simulink model "Modelo_Tanque_Malha_Aberta"  (R2022a)
settings: Solver=FixedStepAuto  StartTime=0.0  StopTime=2500  FixedStep=1e-3  RelTol=1e-3
libraries: simulink x1
settings Model: Creator=User  LastModifiedBy=User
settings DebuggingCC: UnconnectedInputMsg=warning  UnconnectedOutputMsg=warning  UnconnectedLineMsg=warning
settings RTWCC: DLArmComputeVersion=19.05

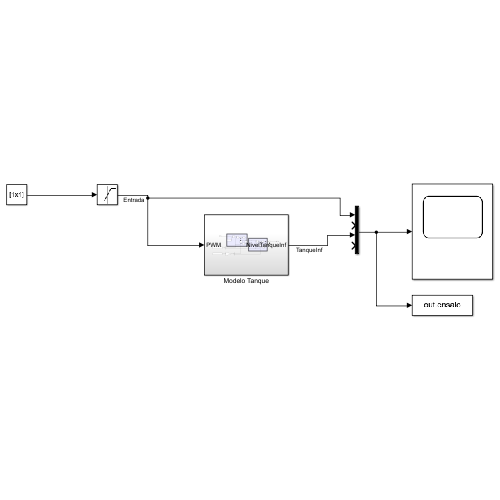
[thumbnail: Simulink's stored preview of the top-level diagram]
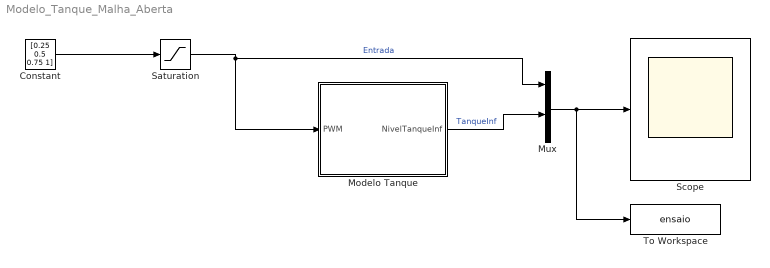
== system Modelo_Tanque_Malha_Aberta ==
  Constant : Constant  Value=[0.25 0.5 0.75 1]
  Modelo Tanque : Subsystem
  Mux : Mux
  Saturation : Saturate  UpperLimit=1  LowerLimit=0
  Scope : Scope
  To Workspace : ToWorkspace  VariableName=ensaio  SaveFormat=Timeseries  SampleTime=40
  wires:
  Saturation/1 -> Modelo Tanque/1(PWM), Mux/1  "Entrada"
  Modelo Tanque/1(NivelTanqueInf) -> Mux/3  "TanqueInf"
  Mux/1 -> To Workspace/1, Scope/1
  Constant/1 -> Saturation/1

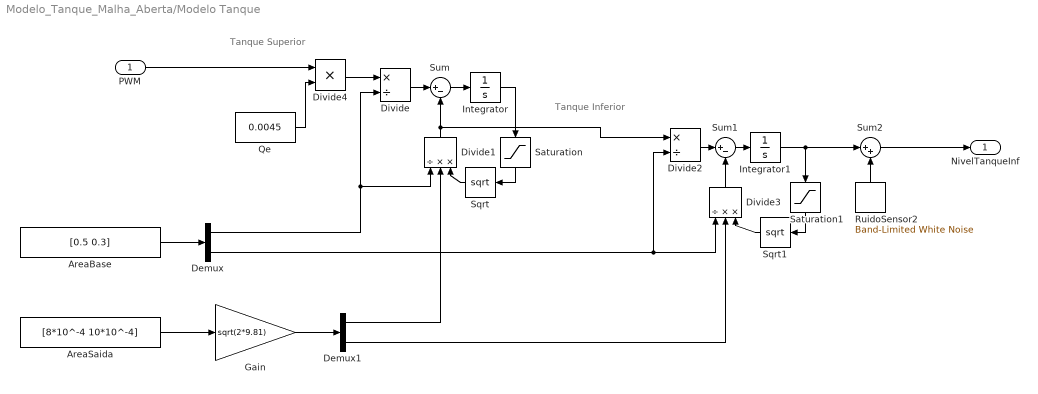
== system Modelo_Tanque_Malha_Aberta/Modelo Tanque ==
  note: Tanque Inferior
  note: Tanque Superior
  PWM : Inport
  AreaBase : Constant  Value=[0.5 0.3]
  AreaSaida : Constant  Value=[8*10^-4 10*10^-4]
  Demux : Demux  Outputs=2
  Demux1 : Demux  Outputs=2
  Divide : Product  Inputs=*/
  Divide1 : Product  Inputs=/**
  Divide2 : Product  Inputs=*/
  Divide3 : Product  Inputs=/**
  Divide4 : Product  Inputs=**
  Gain : Gain  Gain=sqrt(2*9.81)
  Integrator : Integrator
  Integrator1 : Integrator
  Qe : Constant  Value=0.0045
  RuidoSensor2 : simulink/Sources/Band-Limited White Noise  Cov=[0.00001]  Ts=1  seed=[23341]
  Saturation : Saturate  UpperLimit=inf  LowerLimit=0
  Saturation1 : Saturate  UpperLimit=inf  LowerLimit=0
  Sqrt : Sqrt
  Sqrt1 : Sqrt
  Sum : Sum  Inputs=|+-
  Sum1 : Sum  Inputs=|+-
  Sum2 : Sum  Inputs=|++
  NivelTanqueInf : Outport
  wires:
  AreaSaida/1 -> Gain/1
  AreaBase/1 -> Demux/1
  Gain/1 -> Demux1/1
  Integrator/1 -> Saturation/1
  Demux/1 -> Divide/2, Divide1/1
  Divide/1 -> Sum/1
  Sum/1 -> Integrator/1
  Demux1/1 -> Divide1/2
  Sqrt/1 -> Divide1/3
  Integrator1/1 -> Sum2/1, Saturation1/1
  Demux1/2 -> Divide3/2
  Sqrt1/1 -> Divide3/3
  Divide3/1 -> Sum1/2
  Demux/2 -> Divide3/1, Divide2/2
  Sum1/1 -> Integrator1/1
  Divide2/1 -> Sum1/1
  Sum2/1 -> NivelTanqueInf/1
  RuidoSensor2/1 -> Sum2/2
  PWM/1 -> Divide4/1
  Divide1/1 -> Divide2/1, Sum/2
  Saturation/1 -> Sqrt/1
  Saturation1/1 -> Sqrt1/1
  Qe/1 -> Divide4/2
  Divide4/1 -> Divide/1
